simulink model "pr633_phased_detector_loop_filter"  (R2018b)
settings: Solver=VariableStepAuto  StartTime=0.0  StopTime=time_span  RelTol=1e-3  EnableMultiTasking=on
PreLoadFcn:
  | fs=100e6;
  | time_span=32e-6;
settings Model: Creator=GRIHA  LastModifiedBy=Григорий Фокин
settings DataIOCC: LimitDataPoints=on
settings OptimizationCC: LifeSpan=inf
settings DebuggingCC: AllowSymbolicDim=off  SFUnexpectedBacktrackingDiag=warning  SFNoUnconditionalDefaultTransitionDiag=warning  SFExecutionAtInitializationDiag=none
settings ModelReferenceCC: PropagateSignalLabelsOutOfModel=off
settings SFSimCC: SimUseLocalCustomCode=off
settings RTWCC: RTWUseLocalCustomCode=off
settings CodeAppCC: StateflowObjectComments=on
settings GRTTargetCC: TargetLangStandard=C89/C90 (ANSI)
settings ConfigComp: CovMetricSettings=dw  CovHtmlReporting=on  CovSaveCumulativeToWorkspaceVar=on  CovSaveSingleToWorkspaceVar=on  CovExternalEMLEnable=off

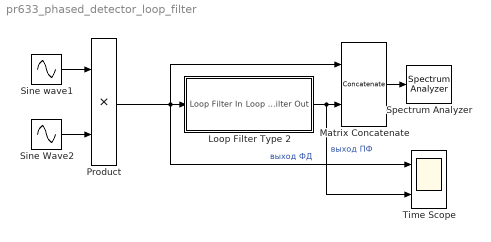
== system pr633_phased_detector_loop_filter ==
  Loop Filter Type 2 : Subsystem  mask{K1=0.03125, K2=1.25e-4}
      mask prompts: K1 "K1 (proportional path)"; K2 "K2 (integral path)"
  Matrix Concatenate : Concatenate  Mode=Multidimensional array  ConcatenateDimension=2
  Product : Product
  Sine Wave2 : Sin  Frequency=2*pi*(fs*1.0/20)  Phase=pi/3  SampleTime=1/fs
  Sine wave1 : Sin  Frequency=2*pi*(fs/20)  SampleTime=1/fs
  Spectrum Analyzer : SpectrumAnalyzer
  Time Scope : Scope  NumInputPorts=2
  wires:
  Sine wave1/1 -> Product/1
  Sine Wave2/1 -> Product/2
  Product/1 -> Loop Filter Type 2/1(Loop Filter In), Matrix Concatenate/1, Time Scope/1  "выход ФД"
  Loop Filter Type 2/1(Loop Filter Out) -> Matrix Concatenate/2, Time Scope/2  "выход ПФ"
  Matrix Concatenate/1 -> Spectrum Analyzer/1

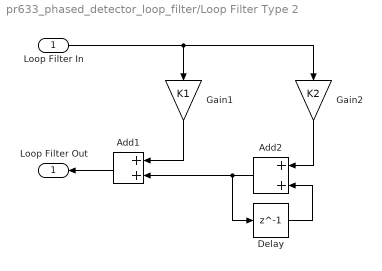
== system pr633_phased_detector_loop_filter/Loop Filter Type 2 ==
  Loop Filter In : Inport
  Add1 : Sum
  Add2 : Sum
  Delay : Delay  DelayLength=1  InitialCondition=0
  Gain1 : Gain  Gain=K1
  Gain2 : Gain  Gain=K2
  Loop Filter Out : Outport
  wires:
  Loop Filter In/1 -> Gain2/1, Gain1/1
  Add1/1 -> Loop Filter Out/1
  Gain1/1 -> Add1/1
  Add2/1 -> Delay/1, Add1/2
  Gain2/1 -> Add2/1
  Delay/1 -> Add2/2
